simulink model "PI_Controller"  (R2020b)
settings: Solver=VariableStepAuto  StartTime=0.0  StopTime=20  RelTol=1e-3
model workspace (MAT data in the model file):
  J = 0.000245
  Kp = 0.3
  ki = 0.2
  ts = 0.01
libraries: simulink x1
settings Model: OrderedModelArguments=off  Creator=dssan  LastModifiedBy=dssan

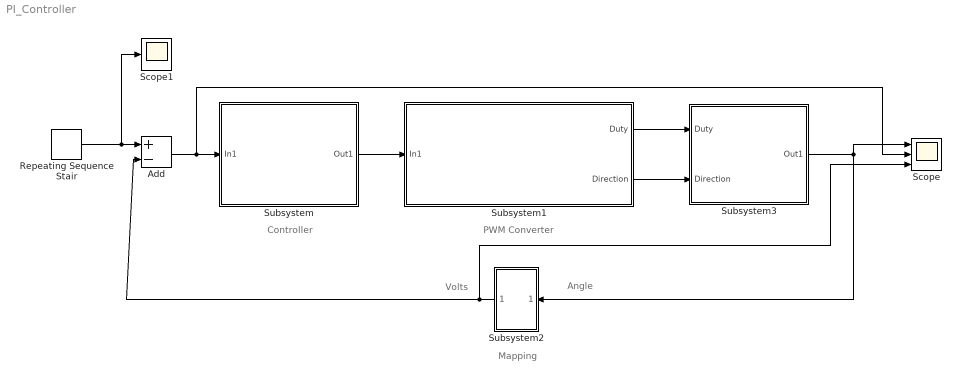
== system PI_Controller ==
  note: Mapping
  note: PWM Converter
  note: Controller
  note: Volts
  note: Angle
  Add : Sum  Inputs=+-
  Repeating Sequence Stair : simulink/Sources/Repeating Sequence Stair  OutValues=[1 2 3 4 5 4 3 2 5].'  tsamp=-1  OutMin=[]  OutMax=[]  OutDataTypeStr=double  OutputDataTypeScalingMode=double  OutDataType=fixdt(0,8)  ConRadixGroup=Best Precision: Vector-wise  OutScaling=2^-12
  Scope : Scope  NumInputPorts=3
  Scope1 : Scope
  Subsystem : Subsystem
  Subsystem1 : Subsystem
  Subsystem2 : Subsystem
  Subsystem3 : Subsystem
  wires:
  Subsystem/1(Out1) -> Subsystem1/1(In1)
  Subsystem2/1(Out1) -> Scope/3, Add/2
  Subsystem3/1(Out1) -> Scope/1, Subsystem2/1(In1)
  Subsystem1/1(Duty) -> Subsystem3/1(Duty)
  Subsystem1/2(Direction) -> Subsystem3/2(Direction)
  Add/1 -> Subsystem/1(In1), Scope/2
  Repeating Sequence Stair/1 -> Scope1/1, Add/1

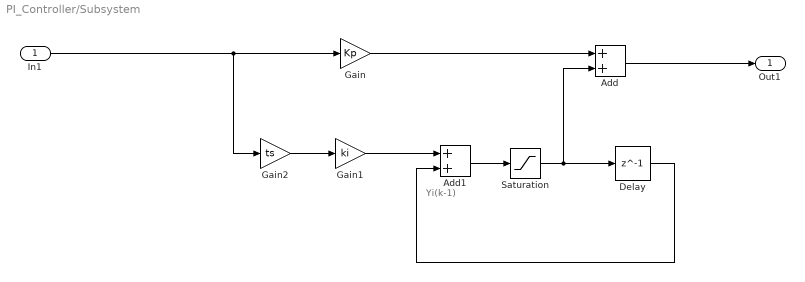
== system PI_Controller/Subsystem ==
  note: Yi(k-1)
  In1 : Inport
  Add : Sum
  Add1 : Sum
  Delay : Delay  DelayLength=1
  Gain : Gain  Gain=Kp
  Gain1 : Gain  Gain=ki
  Gain2 : Gain  Gain=ts
  Saturation : Saturate  UpperLimit=1  LowerLimit=-1
  Out1 : Outport
  wires:
  In1/1 -> Gain2/1, Gain/1
  Delay/1 -> Add1/2
  Add/1 -> Out1/1
  Add1/1 -> Saturation/1
  Gain2/1 -> Gain1/1
  Gain1/1 -> Add1/1
  Gain/1 -> Add/1
  Saturation/1 -> Add/2, Delay/1

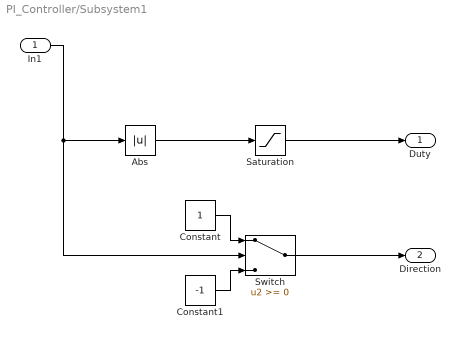
== system PI_Controller/Subsystem1 ==
  In1 : Inport
  Abs : Abs
  Constant : Constant
  Constant1 : Constant  Value=-1
  Saturation : Saturate  UpperLimit=1  LowerLimit=0
  Switch : Switch
  Duty : Outport
  Direction : Outport  Port=2
  wires:
  Abs/1 -> Saturation/1
  In1/1 -> Switch/2, Abs/1
  Constant1/1 -> Switch/3
  Constant/1 -> Switch/1
  Saturation/1 -> Duty/1
  Switch/1 -> Direction/1

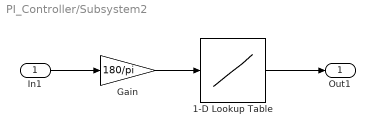
== system PI_Controller/Subsystem2 ==
  In1 : Inport
  1-D Lookup Table : Lookup_n-D  NumberOfTableDimensions=1  BreakpointsForDimension1=[0 90]  Table=[0.5 4.5]  InternalRulePriority=Speed  RndMeth=Simplest  InputSameDT=on
  Gain : Gain  Gain=180/pi
  Out1 : Outport
  wires:
  Gain/1 -> 1-D Lookup Table/1
  In1/1 -> Gain/1
  1-D Lookup Table/1 -> Out1/1

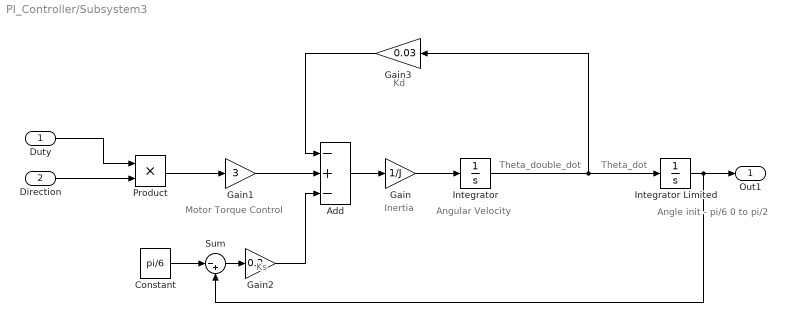
== system PI_Controller/Subsystem3 ==
  note: Theta_dot
  note: Theta_double_dot
  note: Motor Torque Control
  note: Kd
  note: Angle
      | init - pi/6
      | 0 to pi/2
  note: Angular Velocity
  note: Ks
  note: Inertia
  Duty : Inport
  Direction : Inport  Port=2
  Add : Sum  Inputs=-+-
  Constant : Constant  Value=pi/6
  Gain : Gain  Gain=1/J
  Gain1 : Gain  Gain=3
  Gain2 : Gain  Gain=0.2
  Gain3 : Gain  Gain=0.03
  Integrator : Integrator
  Integrator Limited : Integrator  InitialCondition=pi/6  LimitOutput=on  UpperSaturationLimit=pi/2  LowerSaturationLimit=0
  Product : Product
  Sum : Sum  Inputs=|-+
  Out1 : Outport
  wires:
  Sum/1 -> Gain2/1
  Gain2/1 -> Add/3
  Integrator Limited/1 -> Out1/1, Sum/2
  Constant/1 -> Sum/1
  Gain1/1 -> Add/2
  Gain3/1 -> Add/1
  Integrator/1 -> Gain3/1, Integrator Limited/1
  Add/1 -> Gain/1
  Gain/1 -> Integrator/1
  Product/1 -> Gain1/1
  Direction/1 -> Product/2
  Duty/1 -> Product/1
